simulink library "EC2_libraries"  (Simulink 8.9)
settings: Solver=ode1  StartTime=0.0  StopTime=Inf  FixedStep=0.001  RelTol=1e-3  EnableMultiTasking=on
PostLoadFcn:
  | , if any(exist('dsrtsu_mdlpostloadfcn', 'file') == [2, 3, 6]), try dsrtsu_mdlpostloadfcn('Execute', bdroot); catch fprintf('Error in PostLoadFcn (dsrtsu_mdlpostloadfcn) for model "%s":\n %s\n', bdroot, lasterr); end, end,
undefined symbols (not defined in the file): tloop
libraries: EC2_libraries x16, simulink x16, powerlib_extras x1
settings Model: DSRTSU_INTERNAL_RTI_VER=380  DSRTSU_INTERNAL_RTI_TYPE=rti1401  RTICANMMDATA=struct('GeneralSetupData',struct('modelroot',['C:\Temp\WSU\EcoCarII\Controls Repo\PTTR Alpha Branch\Libraries\CAN'],'generalsettings',struct('filesettings',struct('destfolder',struct('Name','RTICANMM_FILES','Check',1),'buildfolder',struct('Name','.','Check',1),'AbsDestfolder',struct('Name',['C:\Temp\WSU\EcoCarII\Controls Repo\PTTR Alpha Branch\Libraries\RTICANMM_FILES']),'AbsBuildfolder',struct('Name',['C:\Temp\WSU\EcoCarII\Controls Repo\PTTR Alpha Branch\Libraries\CAN']))),'options',struct('addpaths',1,'rmpaths',1,'addtrcexclusion',logical(1),'cannavigator',struct('checkmonitoring',0,'serviceno','31','hostservicedefheader',struct('name','x','path','x')),'show_usrtrc',0,'use_usrtrc',0),'advanced',struct('options',[1 1 1 1 1 1 1 1 1 1 1 1 1 1 1 1 1 1 1 1 1 1 1 1 1 1 1 1 1 1 1 1 1 1 1 1 1 1 1 1 1 1 1 1 1 1 1 1 1 1 1 1 1 1 1 1 1 1 1 1 1 1 1 1 1 1 1 1 1 1 1 1 1 1 1 1 1 1 1 1 1 1 1 1 1 1 1 1 1 1 1 1 1 1 1 1 1 1 1 1]),'MPSetup',{{}},'modelname','DIAG_CAN_OUT','block','EC2_libraries'))  Creator=idan  LastModifiedBy=Vraj M

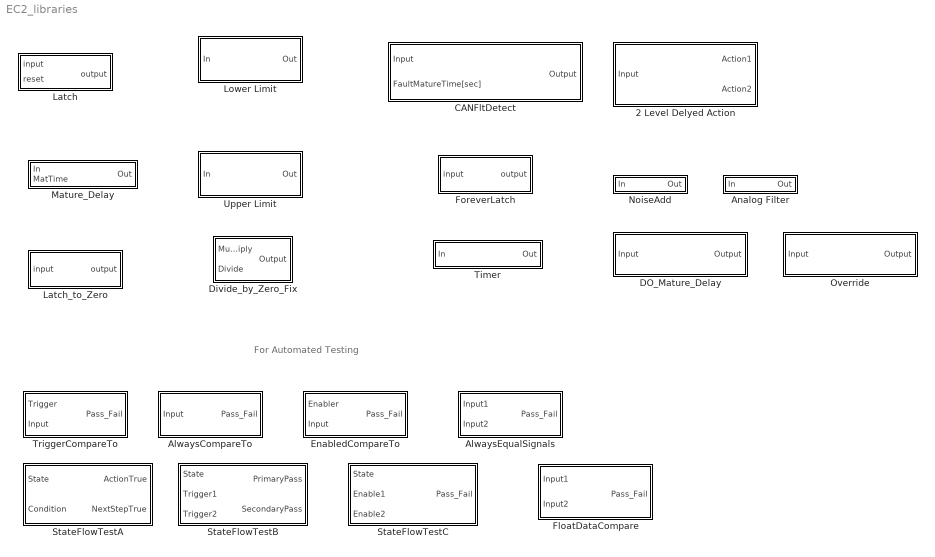
== system EC2_libraries ==
  note: For Automated Testing
  2 Level Delyed Action : Subsystem  mask{LowLimit=0, LowLimitMatureTime=0, HighLimit=0, HighLimitMatureTime=0}
      mask prompts: LowLimit "Low Limit"; LowLimitMatureTime "Low Limit Maturation Time"; HighLimit "High Limit"; HighLimitMatureTime "High Limit Maturation Time"
  AlwaysCompareTo : Subsystem  TreatAsAtomicUnit=on  mask{exp_val=0}
      mask prompts: exp_val "Expected Value"
  AlwaysEqualSignals : Subsystem  TreatAsAtomicUnit=on
  Analog Filter : Subsystem
  CANFltDetect : Subsystem
  DO_Mature_Delay : Subsystem  mask{Time=0}
      mask prompts: Time "DO_Mature_Delay"
  Divide_by_Zero_Fix : Subsystem
  EnabledCompareTo : Subsystem  TreatAsAtomicUnit=on  mask{exp_val=0}
      mask prompts: exp_val "Expected Value"
  FloatDataCompare : Subsystem  mask{Difference=0.001}
  ForeverLatch : Subsystem
  Latch : Subsystem
  Latch_to_Zero : Subsystem
  Lower Limit : Subsystem  mask{Lolimit=0}
      mask prompts: Lolimit "Lower Limit:"
  Mature_Delay : Subsystem
  NoiseAdd : Subsystem  mask{variance=0, seed=0}
  Override : Subsystem  mask{OverrideOn=0, Overide_Value=0}
      mask prompts: OverrideOn "Override_On"; Overide_Value "Override_Value"
  StateFlowTestA : Subsystem  TreatAsAtomicUnit=on  mask{State=2}
      mask prompts: State "First State"
  StateFlowTestB : Subsystem  TreatAsAtomicUnit=on  mask{StateBase=4, PrimaryState=0, SecondaryState=0}
      mask prompts: StateBase "First State"; PrimaryState "Primary State"; SecondaryState "Secondary State"
  StateFlowTestC : Subsystem  TreatAsAtomicUnit=on  mask{StateBase=-4, State=-4}
      mask prompts: StateBase "First State"
  Timer : Subsystem
  TriggerCompareTo : Subsystem  TreatAsAtomicUnit=on  mask{exp_val=0}
      mask prompts: exp_val "Expected Value"
  Upper Limit : Subsystem  mask{Uplimit=0}
      mask prompts: Uplimit "Upper Limit:"

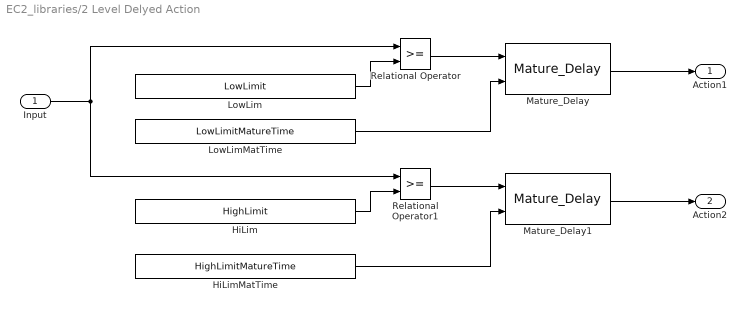
== system EC2_libraries/2 Level Delyed Action ==
  Input : Inport
  HiLim : Constant  Value=HighLimit
  HiLimMatTime : Constant  Value=HighLimitMatureTime
  LowLim : Constant  Value=LowLimit
  LowLimMatTime : Constant  Value=LowLimitMatureTime
  Mature_Delay : EC2_libraries/Mature_Delay
  Mature_Delay1 : EC2_libraries/Mature_Delay
  Relational Operator : RelationalOperator  OutDataTypeStr=boolean  RndMeth=Nearest
  Relational Operator1 : RelationalOperator  OutDataTypeStr=boolean  RndMeth=Nearest
  Action1 : Outport
  Action2 : Outport  Port=2
  wires:
  Input/1 -> Relational Operator/1, Relational Operator1/1
  LowLim/1 -> Relational Operator/2
  Relational Operator/1 -> Mature_Delay/1
  LowLimMatTime/1 -> Mature_Delay/2
  Mature_Delay/1 -> Action1/1
  HiLim/1 -> Relational Operator1/2
  Relational Operator1/1 -> Mature_Delay1/1
  HiLimMatTime/1 -> Mature_Delay1/2
  Mature_Delay1/1 -> Action2/1

== system EC2_libraries/AlwaysCompareTo ==
  Input : Inport
  Compare To Constant13 : simulink/Logic and Bit Operations/Compare To Constant  relop=~=  const=exp_val  OutDataTypeStr=boolean
  Data Type Conversion6 : DataTypeConversion
  Latch_to_Zero6 : EC2_libraries/Latch_to_Zero
  Pass_Fail : Outport
  wires:
  Data Type Conversion6/1 -> Pass_Fail/1
  Latch_to_Zero6/1 -> Data Type Conversion6/1
  Compare To Constant13/1 -> Latch_to_Zero6/1
  Input/1 -> Compare To Constant13/1

== system EC2_libraries/AlwaysEqualSignals ==
  note: Compares the output to ensure always equal to each other
  Input1 : Inport
  Input2 : Inport  Port=2
  Data Type Conversion6 : DataTypeConversion
  Latch_to_Zero6 : EC2_libraries/Latch_to_Zero
  Relational Operator3 : RelationalOperator  Operator=~=  OutDataTypeStr=boolean  RndMeth=Nearest
  Pass_Fail : Outport
  wires:
  Data Type Conversion6/1 -> Pass_Fail/1
  Relational Operator3/1 -> Latch_to_Zero6/1
  Latch_to_Zero6/1 -> Data Type Conversion6/1
  Input2/1 -> Relational Operator3/2
  Input1/1 -> Relational Operator3/1

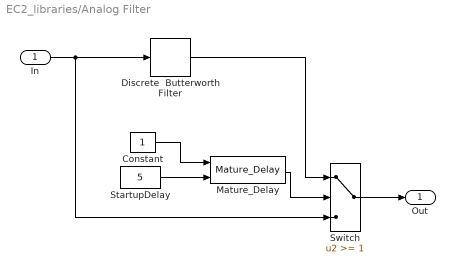
== system EC2_libraries/Analog Filter ==
  In : Inport
  Constant : Constant
  "Discrete  Butterworth Filter " : powerlib_extras/Discrete  Control Blocks/Discrete  Butterworth Filter   SystemSampleTime=-1  FilterType=Lowpass  N=1  Fo=2  Bo=80  Ts=tloop  Initialize=on  Vac_Init=[1.2 60 60]  Vdc_Init=-0.6  PlotResponse=off  param1=[1 500 0.1]
  Mature_Delay : EC2_libraries/Mature_Delay
  StartupDelay : Constant  Value=5
  Switch : Switch  Threshold=1
  Out : Outport
  wires:
  In/1 -> "Discrete  Butterworth Filter "/1, Switch/3
  "Discrete  Butterworth Filter "/1 -> Switch/1
  StartupDelay/1 -> Mature_Delay/2
  Constant/1 -> Mature_Delay/1
  Mature_Delay/1 -> Switch/2
  Switch/1 -> Out/1

== system EC2_libraries/CANFltDetect ==
  Input : Inport
  FaultMatureTime[sec] : Inport  Port=2
  Detect Change : simulink/Logic and Bit Operations/Detect Change  vinit=1  InputProcessing=Inherited  OutDataTypeStr=uint8
  Logical Operator : Logic  Operator=NOT  Inputs=1  AllPortsSameDT=off  OutDataTypeStr=boolean
  Mature_Delay : EC2_libraries/Mature_Delay
  Output : Outport
  wires:
  FaultMatureTime[sec]/1 -> Mature_Delay/2
  Logical Operator/1 -> Mature_Delay/1
  Detect Change/1 -> Logical Operator/1
  Input/1 -> Detect Change/1
  Mature_Delay/1 -> Output/1

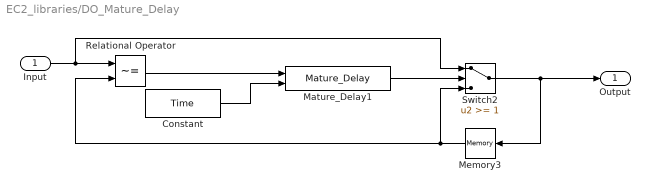
== system EC2_libraries/DO_Mature_Delay ==
  Input : Inport
  Constant : Constant  Value=Time
  Mature_Delay1 : EC2_libraries/Mature_Delay
  Memory3 : Memory
  Relational Operator : RelationalOperator  Operator=~=  OutDataTypeStr=boolean  RndMeth=Nearest
  Switch2 : Switch  Threshold=1
  Output : Outport
  wires:
  Relational Operator/1 -> Mature_Delay1/1
  Constant/1 -> Mature_Delay1/2
  Mature_Delay1/1 -> Switch2/2
  Memory3/1 -> Switch2/3, Relational Operator/2
  Switch2/1 -> Memory3/1, Output/1
  Input/1 -> Relational Operator/1, Switch2/1

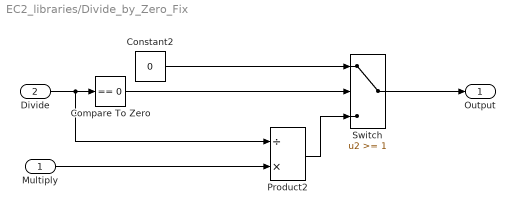
== system EC2_libraries/Divide_by_Zero_Fix ==
  Multiply : Inport
  Divide : Inport  Port=2
  Compare To Zero : simulink/Logic and Bit Operations/Compare To Zero  relop===  OutDataTypeStr=boolean
  Constant2 : Constant  Value=0
  Product2 : Product  Inputs=/*  SaturateOnIntegerOverflow=on  InputSameDT=on  OutDataTypeStr=Inherit: Same as first input
  Switch : Switch  Threshold=1
  Output : Outport
  wires:
  Compare To Zero/1 -> Switch/2
  Constant2/1 -> Switch/1
  Divide/1 -> Compare To Zero/1, Product2/1
  Multiply/1 -> Product2/2
  Switch/1 -> Output/1
  Product2/1 -> Switch/3

== system EC2_libraries/EnabledCompareTo ==
  Enabler : Inport
  Input : Inport  Port=2
  Data Type Conversion6 : DataTypeConversion
  Enabled Subsystem2 : Subsystem  TreatAsAtomicUnit=on
  Latch_to_Zero6 : EC2_libraries/Latch_to_Zero
  Pass_Fail : Outport
  wires:
  Data Type Conversion6/1 -> Pass_Fail/1
  Enabler/1 -> Enabled Subsystem2/Enable
  Enabled Subsystem2/1(Out1) -> Latch_to_Zero6/1
  Latch_to_Zero6/1 -> Data Type Conversion6/1
  Input/1 -> Enabled Subsystem2/1(In1)

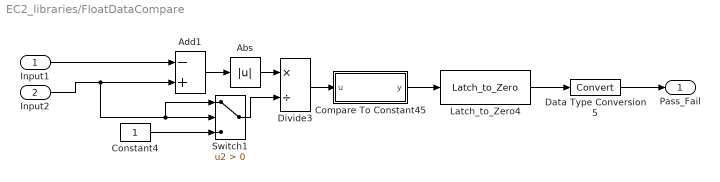
== system EC2_libraries/FloatDataCompare ==
  Input1 : Inport
  Input2 : Inport  Port=2
  Abs : Abs
  Add1 : Sum  Inputs=-+
  Compare To Constant45 : Subsystem  mask(Compare To Constant){relop=>, const=Difference, LogicOutDataTypeMode=boolean, ZeroCross=on}
      mask prompts: relop "Operator:"; const "Constant value:"; LogicOutDataTypeMode "Output data type mode:"; ZeroCross "Enable zero-crossing detection"
      mask help: Determine how a signal compares to a constant.
      mask init:
      | blkName = gcb;
      | 
      | if strcmp(get_param(gcbh,'LogicOutDataTypeMode'),'boolean')
      | 	setValue = 'Boolean';
      | else
      | 	setValue = 'Specify via dialog';
      | end
      | 
      | set_param([blkName,'/Compare'],'relop',relop, ...
      | 	'LogicOutDataTypeMode', setValue, 'ZeroCross', ZeroCross);
      | 
      | str = [relop,' C']; %default
      | 
      | const_str = get_param(blkName, 'const');
      | 
      | if isempty(strfind(const_str, ' ')) && isempty(strfind(const_str, ','))
      |     % scalar or single expression
      |     if isempty(str2num(const_str))
      |         %expression
      |         str = [relop, ' ', const_str];
      |     elseif length(const) == 1
      |         str = [relop,' ',num2str(double(const))];
      |     end
      | end
      mask TypeOptions relop: == | ~= | < | <= | >= | >
      mask TypeOptions LogicOutDataTypeMode: uint8 | boolean
      mask Callback ZeroCross: sl('zeroCrossEnable', gcbh);
      mask Display: disp(str)
  Constant4 : Constant
  Data Type Conversion5 : DataTypeConversion
  Divide3 : Product  Inputs=*/
  Latch_to_Zero4 : EC2_libraries/Latch_to_Zero
  Switch1 : Switch  Criteria=u2 > Threshold
  Pass_Fail : Outport
  wires:
  Input1/1 -> Add1/1
  Divide3/1 -> Compare To Constant45/1(u)
  Abs/1 -> Divide3/1
  Add1/1 -> Abs/1
  Input2/1 -> Switch1/1, Switch1/2, Add1/2
  Compare To Constant45/1(y) -> Latch_to_Zero4/1
  Latch_to_Zero4/1 -> Data Type Conversion5/1
  Switch1/1 -> Divide3/2
  Constant4/1 -> Switch1/3
  Data Type Conversion5/1 -> Pass_Fail/1

== system EC2_libraries/ForeverLatch ==
  input : Inport  OutDataTypeStr=boolean
  Memory : Memory
  OR1 : Logic  Operator=OR  OutDataTypeStr=boolean
  output : Outport  OutDataTypeStr=boolean
  wires:
  OR1/1 -> output/1, Memory/1
  Memory/1 -> OR1/2
  input/1 -> OR1/1

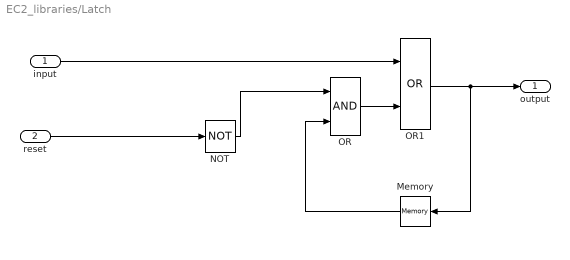
== system EC2_libraries/Latch ==
  input : Inport  OutDataTypeStr=boolean
  reset : Inport  Port=2  OutDataTypeStr=boolean
  Memory : Memory
  NOT : Logic  Operator=NOT  OutDataTypeStr=boolean
  OR : Logic  OutDataTypeStr=boolean
  OR1 : Logic  Operator=OR  OutDataTypeStr=boolean
  output : Outport  OutDataTypeStr=boolean
  wires:
  input/1 -> OR1/1
  reset/1 -> NOT/1
  Memory/1 -> OR/2
  NOT/1 -> OR/1
  OR1/1 -> Memory/1, output/1
  OR/1 -> OR1/2

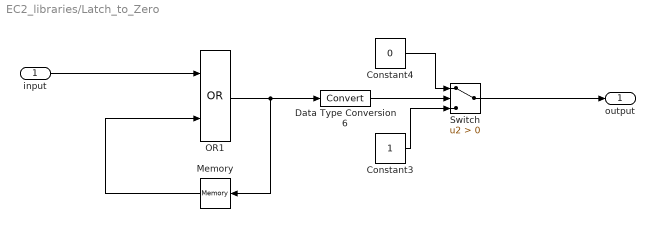
== system EC2_libraries/Latch_to_Zero ==
  input : Inport  OutDataTypeStr=boolean
  Constant3 : Constant
  Constant4 : Constant  Value=0
  Data Type Conversion6 : DataTypeConversion
  Memory : Memory
  OR1 : Logic  Operator=OR  OutDataTypeStr=boolean
  Switch : Switch  Criteria=u2 > Threshold
  output : Outport
  wires:
  Data Type Conversion6/1 -> Switch/2
  input/1 -> OR1/1
  Memory/1 -> OR1/2
  OR1/1 -> Data Type Conversion6/1, Memory/1
  Constant3/1 -> Switch/3
  Constant4/1 -> Switch/1
  Switch/1 -> output/1

== system EC2_libraries/Lower Limit ==
  In : Inport
  Constant : Constant  Value=Lolimit
  MinMax : MinMax  Function=max  Inputs=2
  Out : Outport
  wires:
  MinMax/1 -> Out/1
  In/1 -> MinMax/1
  Constant/1 -> MinMax/2

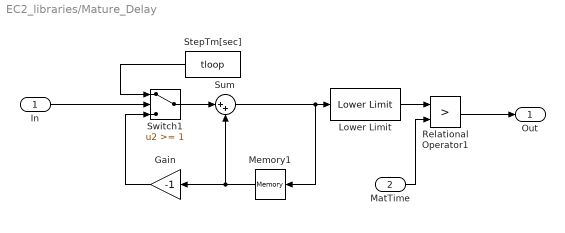
== system EC2_libraries/Mature_Delay ==
  In : Inport
  MatTime : Inport  Port=2
  Gain : Gain  Gain=-1
  Lower Limit : EC2_libraries/Lower Limit  Lolimit=0.001
  Memory1 : Memory
  Relational Operator1 : RelationalOperator  Operator=>  OutDataTypeStr=boolean  RndMeth=Nearest
  StepTm[sec] : Constant  Value=tloop
  Sum : Sum  Inputs=|++
  Switch1 : Switch  Threshold=1
  Out : Outport
  wires:
  In/1 -> Switch1/2
  Gain/1 -> Switch1/3
  Memory1/1 -> Sum/2, Gain/1
  Relational Operator1/1 -> Out/1
  MatTime/1 -> Relational Operator1/2
  StepTm[sec]/1 -> Switch1/1
  Switch1/1 -> Sum/1
  Sum/1 -> Memory1/1, Lower Limit/1
  Lower Limit/1 -> Relational Operator1/1

== system EC2_libraries/NoiseAdd ==
  In : Inport
  Random Number : RandomNumber  Variance=variance  Seed=seed  SampleTime=tloop
  Rate Transition : RateTransition
  Sum : Sum  Inputs=|++
  Out : Outport
  wires:
  Rate Transition/1 -> Sum/2
  Random Number/1 -> Rate Transition/1
  In/1 -> Sum/1
  Sum/1 -> Out/1

== system EC2_libraries/Override ==
  Input : Inport
  Data Type Conversion14 : DataTypeConversion
  OverrideOn : Constant  Value=0
  OverrideValue : Constant  Value=0
  Switch1 : Switch  Threshold=1
  Output : Outport
  wires:
  OverrideOn/1 -> Switch1/2
  OverrideValue/1 -> Switch1/1
  Switch1/1 -> Data Type Conversion14/1
  Input/1 -> Switch1/3
  Data Type Conversion14/1 -> Output/1

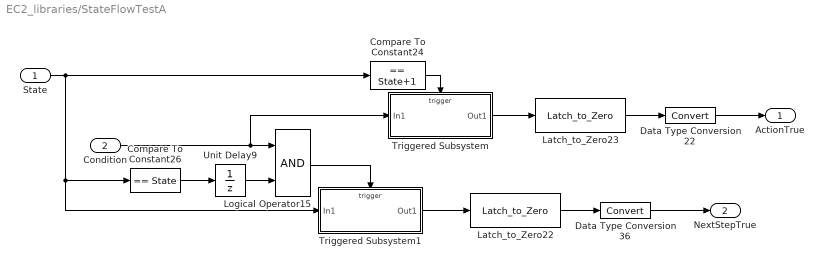
== system EC2_libraries/StateFlowTestA ==
  State : Inport
  Condition : Inport  Port=2
  Compare To Constant24 : simulink/Logic and Bit Operations/Compare To Constant  relop===  const=State+1  OutDataTypeStr=uint8
  Compare To Constant26 : simulink/Logic and Bit Operations/Compare To Constant  relop===  const=State  OutDataTypeStr=uint8
  Data Type Conversion22 : DataTypeConversion
  Data Type Conversion36 : DataTypeConversion
  Latch_to_Zero22 : EC2_libraries/Latch_to_Zero
  Latch_to_Zero23 : EC2_libraries/Latch_to_Zero
  Logical Operator15 : Logic  AllPortsSameDT=off  OutDataTypeStr=boolean
  Triggered Subsystem : Subsystem  TreatAsAtomicUnit=on
  Triggered Subsystem1 : Subsystem  TreatAsAtomicUnit=on
  Unit Delay9 : UnitDelay  SampleTime=-1
  ActionTrue : Outport
  NextStepTrue : Outport  Port=2
  wires:
  Triggered Subsystem1/1(Out1) -> Latch_to_Zero22/1
  Data Type Conversion36/1 -> NextStepTrue/1
  Latch_to_Zero22/1 -> Data Type Conversion36/1
  Triggered Subsystem/1(Out1) -> Latch_to_Zero23/1
  Latch_to_Zero23/1 -> Data Type Conversion22/1
  Compare To Constant24/1 -> Triggered Subsystem/Trigger
  Logical Operator15/1 -> Triggered Subsystem1/Trigger
  State/1 -> Compare To Constant26/1, Triggered Subsystem1/1(In1), Compare To Constant24/1
  Condition/1 -> Logical Operator15/1, Triggered Subsystem/1(In1)
  Compare To Constant26/1 -> Unit Delay9/1
  Unit Delay9/1 -> Logical Operator15/2
  Data Type Conversion22/1 -> ActionTrue/1

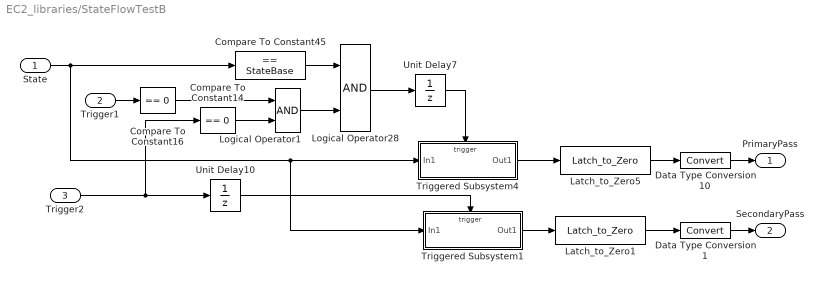
== system EC2_libraries/StateFlowTestB ==
  State : Inport
  Trigger1 : Inport  Port=2
  Trigger2 : Inport  Port=3
  Compare To Constant14 : simulink/Logic and Bit Operations/Compare To Constant  relop===  const=0  OutDataTypeStr=uint8
  Compare To Constant16 : simulink/Logic and Bit Operations/Compare To Constant  relop===  const=0  OutDataTypeStr=uint8
  Compare To Constant45 : simulink/Logic and Bit Operations/Compare To Constant  relop===  const=StateBase  OutDataTypeStr=uint8
  Data Type Conversion1 : DataTypeConversion
  Data Type Conversion10 : DataTypeConversion
  Latch_to_Zero1 : EC2_libraries/Latch_to_Zero
  Latch_to_Zero5 : EC2_libraries/Latch_to_Zero
  Logical Operator1 : Logic  AllPortsSameDT=off  OutDataTypeStr=boolean
  Logical Operator28 : Logic  AllPortsSameDT=off  OutDataTypeStr=boolean
  Triggered Subsystem1 : Subsystem  TreatAsAtomicUnit=on
  Triggered Subsystem4 : Subsystem  TreatAsAtomicUnit=on
  Unit Delay10 : UnitDelay  SampleTime=-1
  Unit Delay7 : UnitDelay  SampleTime=-1
  PrimaryPass : Outport
  SecondaryPass : Outport  Port=2
  wires:
  Unit Delay10/1 -> Triggered Subsystem1/Trigger
  Compare To Constant45/1 -> Logical Operator28/1
  State/1 -> Compare To Constant45/1, Triggered Subsystem1/1(In1), Triggered Subsystem4/1(In1)
  Unit Delay7/1 -> Triggered Subsystem4/Trigger
  Triggered Subsystem4/1(Out1) -> Latch_to_Zero5/1
  Logical Operator28/1 -> Unit Delay7/1
  Triggered Subsystem1/1(Out1) -> Latch_to_Zero1/1
  Compare To Constant16/1 -> Logical Operator1/1
  Logical Operator1/1 -> Logical Operator28/2
  Compare To Constant14/1 -> Logical Operator1/2
  Trigger2/1 -> Unit Delay10/1, Compare To Constant14/1
  Trigger1/1 -> Compare To Constant16/1
  Latch_to_Zero5/1 -> Data Type Conversion10/1
  Latch_to_Zero1/1 -> Data Type Conversion1/1
  Data Type Conversion10/1 -> PrimaryPass/1
  Data Type Conversion1/1 -> SecondaryPass/1

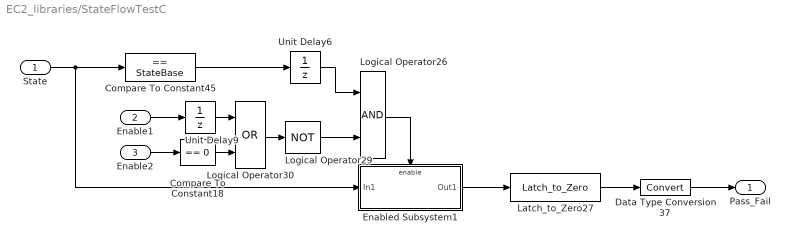
== system EC2_libraries/StateFlowTestC ==
  State : Inport
  Enable1 : Inport  Port=2
  Enable2 : Inport  Port=3
  Compare To Constant18 : simulink/Logic and Bit Operations/Compare To Constant  relop===  const=0  OutDataTypeStr=uint8
  Compare To Constant45 : simulink/Logic and Bit Operations/Compare To Constant  relop===  const=StateBase  OutDataTypeStr=uint8
  Data Type Conversion37 : DataTypeConversion
  Enabled Subsystem1 : Subsystem  TreatAsAtomicUnit=on
  Latch_to_Zero27 : EC2_libraries/Latch_to_Zero
  Logical Operator26 : Logic  AllPortsSameDT=off  OutDataTypeStr=boolean
  Logical Operator29 : Logic  Operator=NOT  AllPortsSameDT=off  OutDataTypeStr=boolean
  Logical Operator30 : Logic  Operator=OR  AllPortsSameDT=off  OutDataTypeStr=boolean
  Unit Delay6 : UnitDelay  SampleTime=-1
  Unit Delay9 : UnitDelay  SampleTime=-1
  Pass_Fail : Outport
  wires:
  Data Type Conversion37/1 -> Pass_Fail/1
  State/1 -> Compare To Constant45/1, Enabled Subsystem1/1(In1)
  Compare To Constant45/1 -> Unit Delay6/1
  Compare To Constant18/1 -> Logical Operator30/2
  Unit Delay9/1 -> Logical Operator30/1
  Unit Delay6/1 -> Logical Operator26/1
  Logical Operator26/1 -> Enabled Subsystem1/Enable
  Logical Operator29/1 -> Logical Operator26/2
  Enable1/1 -> Unit Delay9/1
  Enable2/1 -> Compare To Constant18/1
  Enabled Subsystem1/1(Out1) -> Latch_to_Zero27/1
  Latch_to_Zero27/1 -> Data Type Conversion37/1
  Logical Operator30/1 -> Logical Operator29/1

== system EC2_libraries/Timer ==
  In : Inport
  Gain : Gain  Gain=-1
  Memory1 : Memory
  StepTm[sec] : Constant  Value=tloop
  Sum : Sum  Inputs=|++
  Switch1 : Switch  Threshold=1
  Out : Outport
  wires:
  Memory1/1 -> Sum/2, Gain/1
  StepTm[sec]/1 -> Switch1/1
  Sum/1 -> Memory1/1, Out/1
  Gain/1 -> Switch1/3
  Switch1/1 -> Sum/1
  In/1 -> Switch1/2

== system EC2_libraries/TriggerCompareTo ==
  Trigger : Inport
  Input : Inport  Port=2
  Data Type Conversion6 : DataTypeConversion
  Latch_to_Zero6 : EC2_libraries/Latch_to_Zero
  Triggered Subsystem4 : Subsystem  TreatAsAtomicUnit=on
  Pass_Fail : Outport
  wires:
  Input/1 -> Triggered Subsystem4/1(In1)
  Latch_to_Zero6/1 -> Data Type Conversion6/1
  Triggered Subsystem4/1(Out1) -> Latch_to_Zero6/1
  Trigger/1 -> Triggered Subsystem4/Trigger
  Data Type Conversion6/1 -> Pass_Fail/1

== system EC2_libraries/Upper Limit ==
  In : Inport
  Constant : Constant  Value=Uplimit
  MinMax : MinMax  Inputs=2
  Out : Outport
  wires:
  Constant/1 -> MinMax/2
  In/1 -> MinMax/1
  MinMax/1 -> Out/1

== system EC2_libraries/EnabledCompareTo/Enabled Subsystem2 ==
  In1 : Inport
  Enable : EnablePort
  Compare To Constant1 : simulink/Logic and Bit Operations/Compare To Constant  relop=~=  const=exp_val  OutDataTypeStr=boolean
  Out1 : Outport
  wires:
  Compare To Constant1/1 -> Out1/1
  In1/1 -> Compare To Constant1/1

== system EC2_libraries/FloatDataCompare/Compare To Constant45 ==
  u : Inport
  Compare : RelationalOperator  Operator=>  OutDataTypeStr=boolean  RndMeth=Nearest  InputSameDT=on
  Constant : Constant  DisableCoverage=on  Value=const  OutDataTypeStr=Inherit: Inherit via back propagation
  y : Outport
  wires:
  u/1 -> Compare/1
  Constant/1 -> Compare/2
  Compare/1 -> y/1

== system EC2_libraries/StateFlowTestA/Triggered Subsystem ==
  In1 : Inport
  Trigger : TriggerPort  VariantControl=(inherit)
  Logical Operator18 : Logic  Operator=NOT  AllPortsSameDT=off  OutDataTypeStr=boolean
  Out1 : Outport
  wires:
  In1/1 -> Logical Operator18/1
  Logical Operator18/1 -> Out1/1

== system EC2_libraries/StateFlowTestA/Triggered Subsystem1 ==
  In1 : Inport
  Trigger : TriggerPort  VariantControl=(inherit)
  Compare To Constant : simulink/Logic and Bit Operations/Compare To Constant  relop=~=  const=State+1  OutDataTypeStr=boolean
  Out1 : Outport
  wires:
  In1/1 -> Compare To Constant/1
  Compare To Constant/1 -> Out1/1

== system EC2_libraries/StateFlowTestB/Triggered Subsystem1 ==
  In1 : Inport
  Trigger : TriggerPort  VariantControl=(inherit)
  Compare To Constant13 : simulink/Logic and Bit Operations/Compare To Constant  relop=~=  const=SecondaryState  OutDataTypeStr=boolean
  Out1 : Outport
  wires:
  Compare To Constant13/1 -> Out1/1
  In1/1 -> Compare To Constant13/1

== system EC2_libraries/StateFlowTestB/Triggered Subsystem4 ==
  In1 : Inport
  Trigger : TriggerPort  VariantControl=(inherit)
  Compare To Constant13 : simulink/Logic and Bit Operations/Compare To Constant  relop=~=  const=PrimaryState  OutDataTypeStr=boolean
  Out1 : Outport
  wires:
  Compare To Constant13/1 -> Out1/1
  In1/1 -> Compare To Constant13/1

== system EC2_libraries/StateFlowTestC/Enabled Subsystem1 ==
  In1 : Inport
  Enable : EnablePort
  Compare To Constant13 : simulink/Logic and Bit Operations/Compare To Constant  relop=~=  const=State  OutDataTypeStr=boolean
  Out1 : Outport
  wires:
  Compare To Constant13/1 -> Out1/1
  In1/1 -> Compare To Constant13/1

== system EC2_libraries/TriggerCompareTo/Triggered Subsystem4 ==
  In1 : Inport
  Trigger : TriggerPort  VariantControl=(inherit)
  Compare To Constant13 : simulink/Logic and Bit Operations/Compare To Constant  relop=~=  const=exp_val  OutDataTypeStr=boolean
  Out1 : Outport
  wires:
  In1/1 -> Compare To Constant13/1
  Compare To Constant13/1 -> Out1/1
